simulink model "brine_3_1"  (R2018b)
settings: Solver=VariableStepAuto  StartTime=0.0  StopTime=10.0  RelTol=1e-3
settings Model: Creator=fyna  LastModifiedBy=fyna

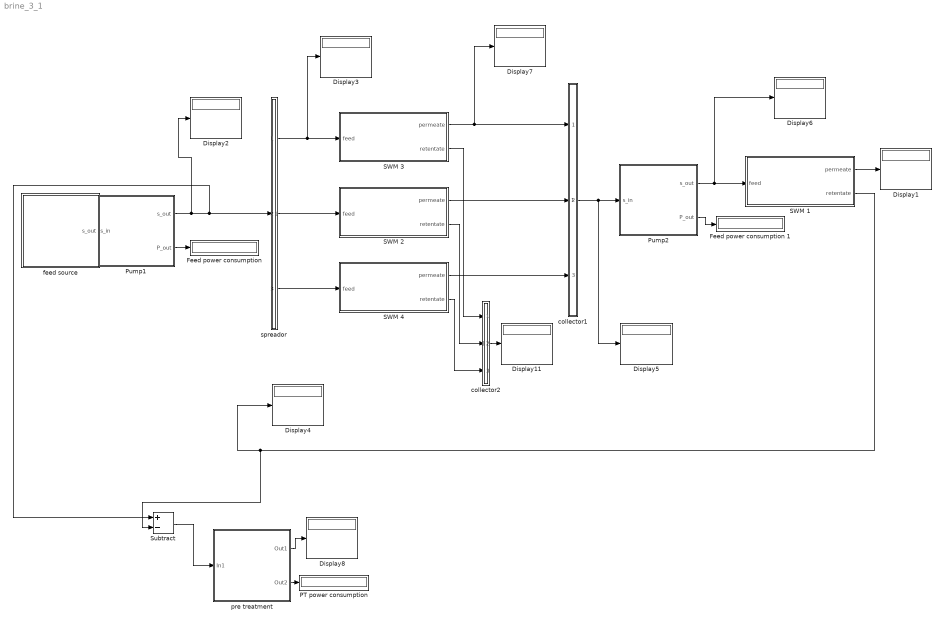
== system brine_3_1 ==
  Display{1..8,11} (9 alike) : Display
  "Feed power consumption " : Display
  Feed power consumption 1 : Display
  "PT power consumption " : Display
  Pump1 : Subsystem  mask(Hydraulic pump){p_f=100, eta=0.8}
      mask prompts: p_f "operating pressure [bar]"; eta "pump efficiency"
      mask help: The hydraulic pump pressurizes the incomming feed stream to the supplied operating pressure. It's power consumption is calculated as P = 3.6e-2*q*p/eta, [P] = kW.
      mask TypeOptions p_f:
      | operating pressure
      | /Value
      mask TypeOptions eta: efficiency/Value
      mask Display: image("pumpSymbol2.png")
  Pump2 : Subsystem  mask(Hydraulic pump){p_f=10, eta=0.8}
      mask prompts: p_f "operating pressure [bar]"; eta "pump efficiency"
      mask help: The hydraulic pump pressurizes the incomming feed stream to the supplied operating pressure. It's power consumption is calculated as P = 3.6e-2*q*p/eta, [P] = kW.
      mask TypeOptions p_f:
      | operating pressure
      | /Value
      mask TypeOptions eta: efficiency/Value
      mask Display: image("pumpSymbol2.png")
  SWM 1 : Subsystem  mask(8040 RO module){waterPerm=5, Value=0.995}
      mask prompts: waterPerm "water permeation coeff [lmh bar]]"; Value "salt rejection"
      mask help:
      | Reverse Osmosis module model. The permeate out-flow and feed out-flow are calculated from their respective in-flows and the membrane characteristics. A 28mil spacer is used in this module type.
      |
      | Input constants: membrane water permeability, salt rejection.
      mask TypeOptions waterPerm: waterPerm/Value
      mask TypeOptions Value: rejectionRate/Value
      mask Display: image('roSymbol.png');
  SWM 2 : Subsystem  mask(8040 RO module){waterPerm=5, Value=0.995}
      mask prompts: waterPerm "water permeation coeff [lmh bar]]"; Value "salt rejection"
      mask help:
      | Reverse Osmosis module model. The permeate out-flow and feed out-flow are calculated from their respective in-flows and the membrane characteristics. A 28mil spacer is used in this module type.
      |
      | Input constants: membrane water permeability, salt rejection.
      mask TypeOptions waterPerm: waterPerm/Value
      mask TypeOptions Value: rejectionRate/Value
      mask Display: image('roSymbol.png');
  SWM 3 : Subsystem  mask(8040 RO module){waterPerm=5, Value=0.995}
      mask prompts: waterPerm "water permeation coeff [lmh bar]]"; Value "salt rejection"
      mask help:
      | Reverse Osmosis module model. The permeate out-flow and feed out-flow are calculated from their respective in-flows and the membrane characteristics. A 28mil spacer is used in this module type.
      |
      | Input constants: membrane water permeability, salt rejection.
      mask TypeOptions waterPerm: waterPerm/Value
      mask TypeOptions Value: rejectionRate/Value
      mask Display: image('roSymbol.png');
  SWM 4 : Subsystem  mask(8040 RO module){waterPerm=5, Value=0.995}
      mask prompts: waterPerm "water permeation coeff [lmh bar]]"; Value "salt rejection"
      mask help:
      | Reverse Osmosis module model. The permeate out-flow and feed out-flow are calculated from their respective in-flows and the membrane characteristics. A 28mil spacer is used in this module type.
      |
      | Input constants: membrane water permeability, salt rejection.
      mask TypeOptions waterPerm: waterPerm/Value
      mask TypeOptions Value: rejectionRate/Value
      mask Display: image('roSymbol.png');
  Subtract : Sum  Inputs=+-
  collector1 : MATLAB Function  TreatAsAtomicUnit=on
  collector2 : MATLAB Function  TreatAsAtomicUnit=on
  feed source : Subsystem  mask(Feed source){Q=1.2e4, p=0, c=1.5}
      mask prompts: Q "flow rate Q [l/h]"; p "pressure p [bar]"; c "concentration c [mol/l]"
      mask help: This element is the starting point for the filtration system.
      mask TypeOptions Q: Q/Value
      mask TypeOptions p: p/Value
      mask TypeOptions c: c/Value
      mask Display: image('sourceSymbol.png');
  "pre treatment " : Subsystem  mask(Pre-treatment element){eta=0.8, k=1, A=100}
      mask prompts: eta "efficiency"; k "PT permeation coeff [m/(d bar)]"; A "PT membr area [m^2]"
      mask help: Simplified pre-treatment model for calculation of power demand only. The incoming stream is transfered to the outlet unchanged. From its flow rate, the pre-treatment pressure and the efficiency the power consumtion is calculated as: P = 3.6e-2*q*p/eta, [P] = kW.
      mask TypeOptions eta: nu/Value
      mask TypeOptions k: permeability const/Value
      mask TypeOptions A: membrSrf/Value
      mask Display: image('ptSymbol.png');
  spreador : MATLAB Function  TreatAsAtomicUnit=on
  wires:
  Pump1/2(P_out) -> "Feed power consumption "/1
  feed source/1(s_out) -> Pump1/1("s_in ")
  SWM 3/2(retentate) -> collector2/1(in_1)
  SWM 1/1(permeate) -> Display1/1
  Pump2/2(P_out) -> Feed power consumption 1/1
  Pump2/1(s_out) -> SWM 1/1(feed), Display6/1
  SWM 1/2(retentate) -> Subtract/2, Display4/1
  Pump1/1(s_out) -> Display2/1, Subtract/1, spreador/1(in_1)
  spreador/1(out_1) -> Display3/1, SWM 3/1(feed)
  spreador/2(data) -> SWM 2/1(feed)
  spreador/3(data1) -> SWM 4/1(feed)
  SWM 2/2(retentate) -> collector2/2(data)
  SWM 4/2(retentate) -> collector2/3(data1)
  SWM 3/1(permeate) -> Display7/1, collector1/1(in_1)
  SWM 4/1(permeate) -> collector1/3(data1)
  SWM 2/1(permeate) -> collector1/2(data)
  collector1/1(out_1) -> Pump2/1("s_in "), Display5/1
  collector2/1(out_1) -> Display11/1
  "pre treatment "/2(Out2) -> "PT power consumption "/1
  Subtract/1 -> "pre treatment "/1(In1)
  "pre treatment "/1(Out1) -> Display8/1

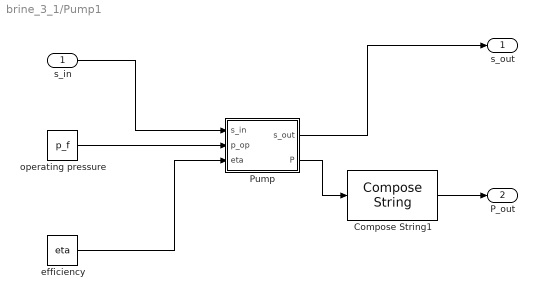
== system brine_3_1/Pump1 ==
  "s_in " : Inport
  Compose String1 : ComposeString  Format='P = %.3f kW'
  Pump : MATLAB Function  TreatAsAtomicUnit=on
  efficiency : Constant  Value=eta
  "operating pressure " : Constant  Value=p_f
  s_out : Outport
  P_out : Outport  Port=2
  wires:
  Pump/1(s_out) -> s_out/1
  efficiency/1 -> Pump/3(eta)
  Compose String1/1 -> P_out/1
  Pump/2(P) -> Compose String1/1
  "s_in "/1 -> Pump/1(s_in)
  "operating pressure "/1 -> Pump/2(p_op)

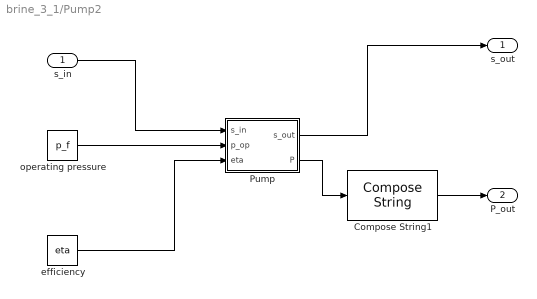
== system brine_3_1/Pump2 ==
  "s_in " : Inport
  Compose String1 : ComposeString  Format='P = %.3f kW'
  Pump : MATLAB Function  TreatAsAtomicUnit=on
  efficiency : Constant  Value=eta
  "operating pressure " : Constant  Value=p_f
  s_out : Outport
  P_out : Outport  Port=2
  wires:
  Pump/1(s_out) -> s_out/1
  efficiency/1 -> Pump/3(eta)
  Compose String1/1 -> P_out/1
  Pump/2(P) -> Compose String1/1
  "s_in "/1 -> Pump/1(s_in)
  "operating pressure "/1 -> Pump/2(p_op)

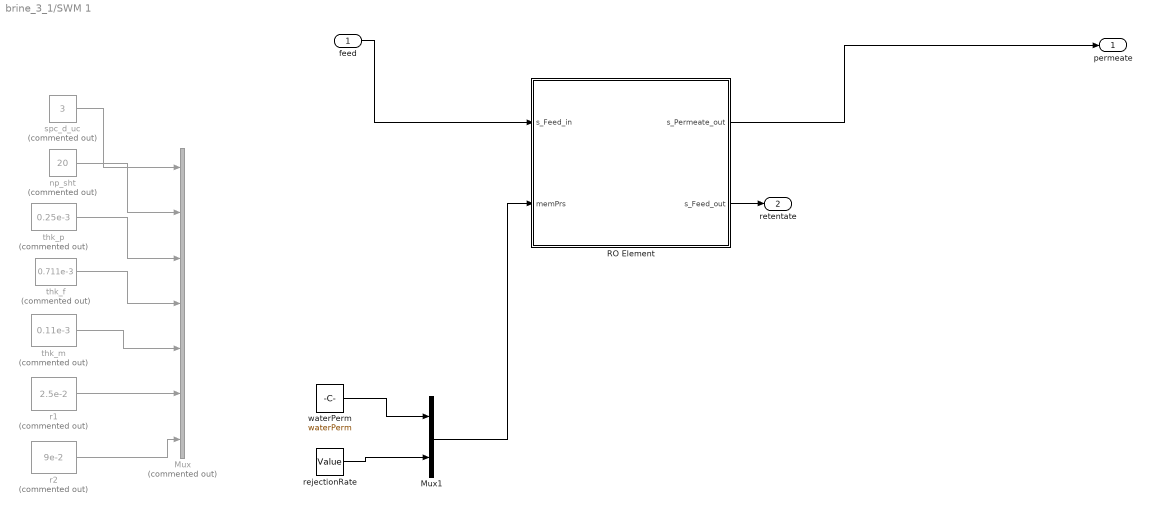
== system brine_3_1/SWM 1 ==
  feed : Inport
  Mux : Mux  Commented=on  Inputs=7
  Mux1 : Mux  Inputs=2
  RO Element : MATLAB Function  TreatAsAtomicUnit=on
  np_sht : Constant  Commented=on  Value=20
  r1 : Constant  Commented=on  Value=2.5e-2
  r2 : Constant  Commented=on  Value=9e-2
  rejectionRate : Constant  Value=Value
  spc_d_uc : Constant  Commented=on  Value=3
  thk_f : Constant  Commented=on  Value=0.711e-3
  thk_m : Constant  Commented=on  Value=0.11e-3
  thk_p : Constant  Commented=on  Value=0.25e-3
  waterPerm : Constant  Value=waterPerm
  permeate : Outport
  retentate : Outport  Port=2
  wires:
  spc_d_uc/1 -> Mux/1
  feed/1 -> RO Element/1(s_Feed_in)
  waterPerm/1 -> Mux1/1
  r1/1 -> Mux/6
  thk_m/1 -> Mux/5
  Mux1/1 -> RO Element/2(memPrs)
  r2/1 -> Mux/7
  RO Element/2(s_Feed_out) -> retentate/1
  rejectionRate/1 -> Mux1/2
  RO Element/1(s_Permeate_out) -> permeate/1
  thk_p/1 -> Mux/3
  thk_f/1 -> Mux/4
  np_sht/1 -> Mux/2

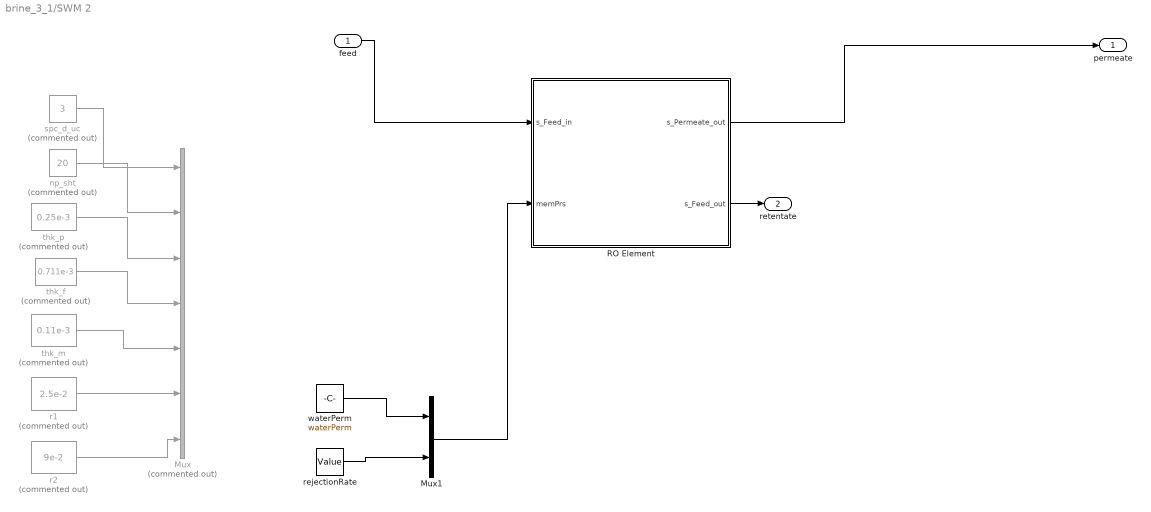
== system brine_3_1/SWM 2 ==
  feed : Inport
  Mux : Mux  Commented=on  Inputs=7
  Mux1 : Mux  Inputs=2
  RO Element : MATLAB Function  TreatAsAtomicUnit=on
  np_sht : Constant  Commented=on  Value=20
  r1 : Constant  Commented=on  Value=2.5e-2
  r2 : Constant  Commented=on  Value=9e-2
  rejectionRate : Constant  Value=Value
  spc_d_uc : Constant  Commented=on  Value=3
  thk_f : Constant  Commented=on  Value=0.711e-3
  thk_m : Constant  Commented=on  Value=0.11e-3
  thk_p : Constant  Commented=on  Value=0.25e-3
  waterPerm : Constant  Value=waterPerm
  permeate : Outport
  retentate : Outport  Port=2
  wires:
  spc_d_uc/1 -> Mux/1
  feed/1 -> RO Element/1(s_Feed_in)
  waterPerm/1 -> Mux1/1
  r1/1 -> Mux/6
  thk_m/1 -> Mux/5
  Mux1/1 -> RO Element/2(memPrs)
  r2/1 -> Mux/7
  RO Element/2(s_Feed_out) -> retentate/1
  rejectionRate/1 -> Mux1/2
  RO Element/1(s_Permeate_out) -> permeate/1
  thk_p/1 -> Mux/3
  thk_f/1 -> Mux/4
  np_sht/1 -> Mux/2

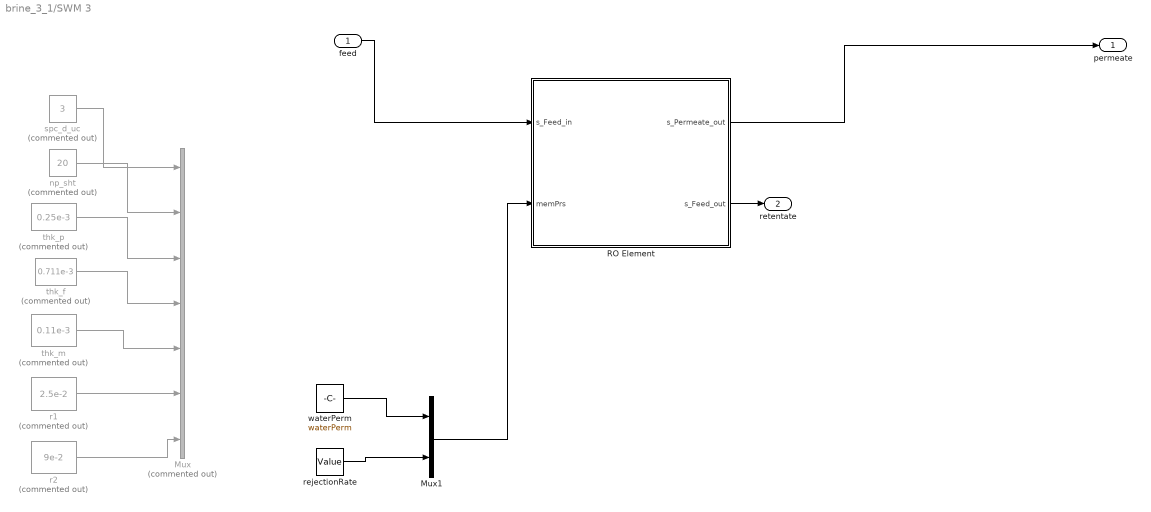
== system brine_3_1/SWM 3 ==
  feed : Inport
  Mux : Mux  Commented=on  Inputs=7
  Mux1 : Mux  Inputs=2
  RO Element : MATLAB Function  TreatAsAtomicUnit=on
  np_sht : Constant  Commented=on  Value=20
  r1 : Constant  Commented=on  Value=2.5e-2
  r2 : Constant  Commented=on  Value=9e-2
  rejectionRate : Constant  Value=Value
  spc_d_uc : Constant  Commented=on  Value=3
  thk_f : Constant  Commented=on  Value=0.711e-3
  thk_m : Constant  Commented=on  Value=0.11e-3
  thk_p : Constant  Commented=on  Value=0.25e-3
  waterPerm : Constant  Value=waterPerm
  permeate : Outport
  retentate : Outport  Port=2
  wires:
  spc_d_uc/1 -> Mux/1
  feed/1 -> RO Element/1(s_Feed_in)
  waterPerm/1 -> Mux1/1
  r1/1 -> Mux/6
  thk_m/1 -> Mux/5
  Mux1/1 -> RO Element/2(memPrs)
  r2/1 -> Mux/7
  RO Element/2(s_Feed_out) -> retentate/1
  rejectionRate/1 -> Mux1/2
  RO Element/1(s_Permeate_out) -> permeate/1
  thk_p/1 -> Mux/3
  thk_f/1 -> Mux/4
  np_sht/1 -> Mux/2

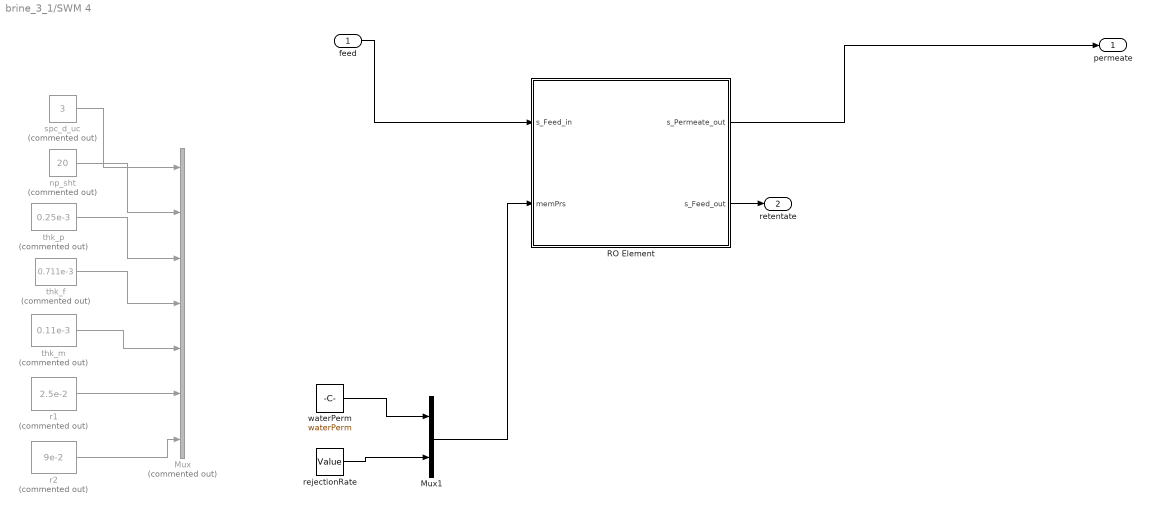
== system brine_3_1/SWM 4 ==
  feed : Inport
  Mux : Mux  Commented=on  Inputs=7
  Mux1 : Mux  Inputs=2
  RO Element : MATLAB Function  TreatAsAtomicUnit=on
  np_sht : Constant  Commented=on  Value=20
  r1 : Constant  Commented=on  Value=2.5e-2
  r2 : Constant  Commented=on  Value=9e-2
  rejectionRate : Constant  Value=Value
  spc_d_uc : Constant  Commented=on  Value=3
  thk_f : Constant  Commented=on  Value=0.711e-3
  thk_m : Constant  Commented=on  Value=0.11e-3
  thk_p : Constant  Commented=on  Value=0.25e-3
  waterPerm : Constant  Value=waterPerm
  permeate : Outport
  retentate : Outport  Port=2
  wires:
  spc_d_uc/1 -> Mux/1
  feed/1 -> RO Element/1(s_Feed_in)
  waterPerm/1 -> Mux1/1
  r1/1 -> Mux/6
  thk_m/1 -> Mux/5
  Mux1/1 -> RO Element/2(memPrs)
  r2/1 -> Mux/7
  RO Element/2(s_Feed_out) -> retentate/1
  rejectionRate/1 -> Mux1/2
  RO Element/1(s_Permeate_out) -> permeate/1
  thk_p/1 -> Mux/3
  thk_f/1 -> Mux/4
  np_sht/1 -> Mux/2

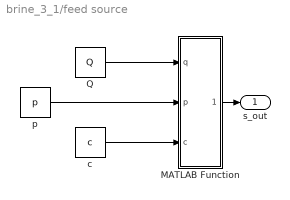
== system brine_3_1/feed source ==
  MATLAB Function : MATLAB Function  TreatAsAtomicUnit=on
  Q : Constant  Value=Q
  c : Constant  Value=c
  p : Constant  Value=p
  s_out : Outport
  wires:
  MATLAB Function/1(s_out) -> s_out/1
  c/1 -> MATLAB Function/3(c)
  p/1 -> MATLAB Function/2(p)
  Q/1 -> MATLAB Function/1(q)

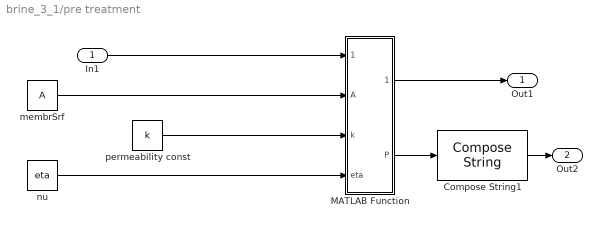
== system brine_3_1/pre treatment  ==
  In1 : Inport
  Compose String1 : ComposeString  Format='P = %.3f kW'
  MATLAB Function : MATLAB Function  TreatAsAtomicUnit=on
  membrSrf : Constant  Value=A
  nu : Constant  Value=eta
  permeability const : Constant  Value=k
  Out1 : Outport
  Out2 : Outport  Port=2
  wires:
  MATLAB Function/1(s_out) -> Out1/1
  In1/1 -> MATLAB Function/1(s_in)
  membrSrf/1 -> MATLAB Function/2(A)
  nu/1 -> MATLAB Function/4(eta)
  MATLAB Function/2(P) -> Compose String1/1
  Compose String1/1 -> Out2/1
  permeability const/1 -> MATLAB Function/3(k)

== matlab function brine_3_1/SWM 1/RO Element ==
  data: s_Feed_in input; s_Permeate_out output; s_Feed_out output; memPrs input
function [s_Permeate_out, s_Feed_out] = fcn(s_Feed_in, memPrs)

% moduleParas = [d_uc, no_sht, thk_d, thk_f, thk_m, r1, r2]

r_fl    = 2.5e-4;
h_ch    = 7.11e-4;
l_f     = 2.822e-3;
eps     = 1.0 - (3.14*r_fl^2*2.0)/(l_f*h_ch);

% ---------------------------------fixing flow rate:
nbSheets = 20;
l_s     = 1.1;
l_l     = 0.93;

q_in    = s_Feed_in(1)/3.6*1e-6;        %m^3/s
U       = q_in/(l_s*0.711e-3*nbSheets);

dh      = 1.0673e-3;        % m
re      = U*dh*1e6;
% sh      = 4.43655*re^0.48267

k_dc    = 1.654*(2.0*r_fl/h_ch)^-0.039*eps^0.75*0.7071^0.086;
sc      = 690;
sh     = 0.664*k_dc*re^0.5*sc^0.33*(dh/l_f)^0.5;

D       = 1.45e-9;          % m^2/s
k_m     = sh*D/dh;        

A_m     = memPrs(1)/3.6*1e-11;  % m/s/pa
zeta    = 8.05e4;               % pa m^3/kg
molarMassNaCl   = 58.44276;     % g/mol
c_f     = s_Feed_in(3)*molarMassNaCl;       %g/l
d_p     = s_Feed_in(2)*1e5;  % pa

a   = 0.0;
b   = 1e-4;

presDiff = d_p - c_f*zeta;
if presDiff > 0
    %fprintf('pi_f = %e, p_f = %e\n',c_f*zeta, d_p);
    jw_uc   = 0.0;
    while abs(a-b) > 1e-10
        x   = 0.5*(a+b);
        fa  = a - A_m*(  d_p - zeta*( c_f*exp(a/k_m) )  );
        fx  = x - A_m*(  d_p - zeta*( c_f*exp(x/k_m) )  );
%         fprintf('a = %e, b = %e, x = %e, abs(a-b) = %e\n',a,b,x, abs(a-b));

        if fa*fx>0
            a   = x;
        else
            b   = x;
        end
    end
    jw_uc   = 0.5*(a+b);
else
    fprintf('osmotic pressure higher than feed hydraulic pressure: pi_f = %e, p_f = %e\n',c_f*zeta, d_p);
    jw_uc   = 0.0;
end

% fprintf('jw = %e\n',jw_uc);
% n_s = round(l_s/(2.822e-3));
% n_l = round(l_l/(2.822e-3));
% area_uc = 16e-6;                %m^2
% area_mod = area_uc*n_s*n_l*nbSheets

area_mod = l_s*l_l*2*nbSheets;

q_mem = area_mod*jw_uc;         % m^3/s
if q_mem > q_in
    q_mem = q_in;
end

% ---------------------------------fixing solute flux:
R_m   = memPrs(2);
q_s_m = q_mem*c_f*(1.0-R_m);    % kg/m^3, solute mass flow rate through membrane
q_s_r = (q_in*c_f - q_s_m);     % kg/m^3, solute mass flow rate retained in feed channel

% ---------------------------------fixing pressure drop:
% f       = 22.91*re^-0.606
f      = 6.23*re^-0.3;
dP      = f*U^2*1e3*l_l/(2.0*dh)*1e-5;  % bar
% fprintf('f = %e\n',area_mod);

q_feed_out = (q_in-q_mem)*3.6e6 ;
p_feed_out = s_Feed_in(2) - dP;q_perm_out = q_mem*3.6e6;      %l/h
c_feed_out = q_s_r/(q_feed_out/3.6e6)/molarMassNaCl;

q_perm_out = q_mem*3.6e6;      %l/h
p_perm_out = 0;

if q_mem > 0
    c_perm_out =  q_s_m/q_mem/molarMassNaCl;
else
    c_perm_out = 0;
end

s_Feed_out      = [q_feed_out, p_feed_out, c_feed_out];
s_Permeate_out  = [q_perm_out, p_perm_out, c_perm_out];

== matlab function brine_3_1/Pump2/Pump ==
  data: s_in input; p_op input; s_out output; eta input; P output
function [s_out,P ] = fcn(s_in, p_op, eta)
q = s_in(1);
dp = p_op - s_in(2);
P = q*dp/eta/3.6e4;     % power consumption in kW
s_out = [q,p_op,s_in(3)];

== matlab function brine_3_1/Pump1/Pump ==
  data: s_in input; p_op input; s_out output; eta input; P output
function [s_out,P ] = fcn(s_in, p_op, eta)
q = s_in(1);
dp = p_op - s_in(2);
P = q*dp/eta/3.6e4;     % power consumption in kW
s_out = [q,p_op,s_in(3)];

== matlab function brine_3_1/SWM 3/RO Element ==
  data: s_Feed_in input; s_Permeate_out output; s_Feed_out output; memPrs input
function [s_Permeate_out, s_Feed_out] = fcn(s_Feed_in, memPrs)

% moduleParas = [d_uc, no_sht, thk_d, thk_f, thk_m, r1, r2]

r_fl    = 2.5e-4;
h_ch    = 7.11e-4;
l_f     = 2.822e-3;
eps     = 1.0 - (3.14*r_fl^2*2.0)/(l_f*h_ch);

% ---------------------------------fixing flow rate:
nbSheets = 20;
l_s     = 1.1;
l_l     = 0.93;

q_in    = s_Feed_in(1)/3.6*1e-6;        %m^3/s
U       = q_in/(l_s*0.711e-3*nbSheets);

dh      = 1.0673e-3;        % m
re      = U*dh*1e6;
% sh      = 4.43655*re^0.48267

k_dc    = 1.654*(2.0*r_fl/h_ch)^-0.039*eps^0.75*0.7071^0.086;
sc      = 690;
sh     = 0.664*k_dc*re^0.5*sc^0.33*(dh/l_f)^0.5;

D       = 1.45e-9;          % m^2/s
k_m     = sh*D/dh;        

A_m     = memPrs(1)/3.6*1e-11;  % m/s/pa
zeta    = 8.05e4;               % pa m^3/kg
molarMassNaCl   = 58.44276;     % g/mol
c_f     = s_Feed_in(3)*molarMassNaCl;       %g/l
d_p     = s_Feed_in(2)*1e5;  % pa

a   = 0.0;
b   = 1e-4;

presDiff = d_p - c_f*zeta;
if presDiff > 0
    %fprintf('pi_f = %e, p_f = %e\n',c_f*zeta, d_p);
    jw_uc   = 0.0;
    while abs(a-b) > 1e-10
        x   = 0.5*(a+b);
        fa  = a - A_m*(  d_p - zeta*( c_f*exp(a/k_m) )  );
        fx  = x - A_m*(  d_p - zeta*( c_f*exp(x/k_m) )  );
%         fprintf('a = %e, b = %e, x = %e, abs(a-b) = %e\n',a,b,x, abs(a-b));

        if fa*fx>0
            a   = x;
        else
            b   = x;
        end
    end
    jw_uc   = 0.5*(a+b);
else
    fprintf('osmotic pressure higher than feed hydraulic pressure: pi_f = %e, p_f = %e\n',c_f*zeta, d_p);
    jw_uc   = 0.0;
end

% fprintf('jw = %e\n',jw_uc);
% n_s = round(l_s/(2.822e-3));
% n_l = round(l_l/(2.822e-3));
% area_uc = 16e-6;                %m^2
% area_mod = area_uc*n_s*n_l*nbSheets

area_mod = l_s*l_l*2*nbSheets;

q_mem = area_mod*jw_uc;         % m^3/s
if q_mem > q_in
    q_mem = q_in;
end

% ---------------------------------fixing solute flux:
R_m   = memPrs(2);
q_s_m = q_mem*c_f*(1.0-R_m);    % kg/m^3, solute mass flow rate through membrane
q_s_r = (q_in*c_f - q_s_m);     % kg/m^3, solute mass flow rate retained in feed channel

% ---------------------------------fixing pressure drop:
% f       = 22.91*re^-0.606
f      = 6.23*re^-0.3;
dP      = f*U^2*1e3*l_l/(2.0*dh)*1e-5;  % bar
% fprintf('f = %e\n',area_mod);

q_feed_out = (q_in-q_mem)*3.6e6 ;
p_feed_out = s_Feed_in(2) - dP;q_perm_out = q_mem*3.6e6;      %l/h
c_feed_out = q_s_r/(q_feed_out/3.6e6)/molarMassNaCl;

q_perm_out = q_mem*3.6e6;      %l/h
p_perm_out = 0;

if q_mem > 0
    c_perm_out =  q_s_m/q_mem/molarMassNaCl;
else
    c_perm_out = 0;
end

s_Feed_out      = [q_feed_out, p_feed_out, c_feed_out];
s_Permeate_out  = [q_perm_out, p_perm_out, c_perm_out];

== matlab function brine_3_1/SWM 2/RO Element ==
  data: s_Feed_in input; s_Permeate_out output; s_Feed_out output; memPrs input
function [s_Permeate_out, s_Feed_out] = fcn(s_Feed_in, memPrs)

% moduleParas = [d_uc, no_sht, thk_d, thk_f, thk_m, r1, r2]

r_fl    = 2.5e-4;
h_ch    = 7.11e-4;
l_f     = 2.822e-3;
eps     = 1.0 - (3.14*r_fl^2*2.0)/(l_f*h_ch);

% ---------------------------------fixing flow rate:
nbSheets = 20;
l_s     = 1.1;
l_l     = 0.93;

q_in    = s_Feed_in(1)/3.6*1e-6;        %m^3/s
U       = q_in/(l_s*0.711e-3*nbSheets);

dh      = 1.0673e-3;        % m
re      = U*dh*1e6;
% sh      = 4.43655*re^0.48267

k_dc    = 1.654*(2.0*r_fl/h_ch)^-0.039*eps^0.75*0.7071^0.086;
sc      = 690;
sh     = 0.664*k_dc*re^0.5*sc^0.33*(dh/l_f)^0.5;

D       = 1.45e-9;          % m^2/s
k_m     = sh*D/dh;        

A_m     = memPrs(1)/3.6*1e-11;  % m/s/pa
zeta    = 8.05e4;               % pa m^3/kg
molarMassNaCl   = 58.44276;     % g/mol
c_f     = s_Feed_in(3)*molarMassNaCl;       %g/l
d_p     = s_Feed_in(2)*1e5;  % pa

a   = 0.0;
b   = 1e-4;

presDiff = d_p - c_f*zeta;
if presDiff > 0
    %fprintf('pi_f = %e, p_f = %e\n',c_f*zeta, d_p);
    jw_uc   = 0.0;
    while abs(a-b) > 1e-10
        x   = 0.5*(a+b);
        fa  = a - A_m*(  d_p - zeta*( c_f*exp(a/k_m) )  );
        fx  = x - A_m*(  d_p - zeta*( c_f*exp(x/k_m) )  );
%         fprintf('a = %e, b = %e, x = %e, abs(a-b) = %e\n',a,b,x, abs(a-b));

        if fa*fx>0
            a   = x;
        else
            b   = x;
        end
    end
    jw_uc   = 0.5*(a+b);
else
    fprintf('osmotic pressure higher than feed hydraulic pressure: pi_f = %e, p_f = %e\n',c_f*zeta, d_p);
    jw_uc   = 0.0;
end

% fprintf('jw = %e\n',jw_uc);
% n_s = round(l_s/(2.822e-3));
% n_l = round(l_l/(2.822e-3));
% area_uc = 16e-6;                %m^2
% area_mod = area_uc*n_s*n_l*nbSheets

area_mod = l_s*l_l*2*nbSheets;

q_mem = area_mod*jw_uc;         % m^3/s
if q_mem > q_in
    q_mem = q_in;
end

% ---------------------------------fixing solute flux:
R_m   = memPrs(2);
q_s_m = q_mem*c_f*(1.0-R_m);    % kg/m^3, solute mass flow rate through membrane
q_s_r = (q_in*c_f - q_s_m);     % kg/m^3, solute mass flow rate retained in feed channel

% ---------------------------------fixing pressure drop:
% f       = 22.91*re^-0.606
f      = 6.23*re^-0.3;
dP      = f*U^2*1e3*l_l/(2.0*dh)*1e-5;  % bar
% fprintf('f = %e\n',area_mod);

q_feed_out = (q_in-q_mem)*3.6e6 ;
p_feed_out = s_Feed_in(2) - dP;q_perm_out = q_mem*3.6e6;      %l/h
c_feed_out = q_s_r/(q_feed_out/3.6e6)/molarMassNaCl;

q_perm_out = q_mem*3.6e6;      %l/h
p_perm_out = 0;

if q_mem > 0
    c_perm_out =  q_s_m/q_mem/molarMassNaCl;
else
    c_perm_out = 0;
end

s_Feed_out      = [q_feed_out, p_feed_out, c_feed_out];
s_Permeate_out  = [q_perm_out, p_perm_out, c_perm_out];

== matlab function brine_3_1/SWM 4/RO Element ==
  data: s_Feed_in input; s_Permeate_out output; s_Feed_out output; memPrs input
function [s_Permeate_out, s_Feed_out] = fcn(s_Feed_in, memPrs)

% moduleParas = [d_uc, no_sht, thk_d, thk_f, thk_m, r1, r2]

r_fl    = 2.5e-4;
h_ch    = 7.11e-4;
l_f     = 2.822e-3;
eps     = 1.0 - (3.14*r_fl^2*2.0)/(l_f*h_ch);

% ---------------------------------fixing flow rate:
nbSheets = 20;
l_s     = 1.1;
l_l     = 0.93;

q_in    = s_Feed_in(1)/3.6*1e-6;        %m^3/s
U       = q_in/(l_s*0.711e-3*nbSheets);

dh      = 1.0673e-3;        % m
re      = U*dh*1e6;
% sh      = 4.43655*re^0.48267

k_dc    = 1.654*(2.0*r_fl/h_ch)^-0.039*eps^0.75*0.7071^0.086;
sc      = 690;
sh     = 0.664*k_dc*re^0.5*sc^0.33*(dh/l_f)^0.5;

D       = 1.45e-9;          % m^2/s
k_m     = sh*D/dh;        

A_m     = memPrs(1)/3.6*1e-11;  % m/s/pa
zeta    = 8.05e4;               % pa m^3/kg
molarMassNaCl   = 58.44276;     % g/mol
c_f     = s_Feed_in(3)*molarMassNaCl;       %g/l
d_p     = s_Feed_in(2)*1e5;  % pa

a   = 0.0;
b   = 1e-4;

presDiff = d_p - c_f*zeta;
if presDiff > 0
    %fprintf('pi_f = %e, p_f = %e\n',c_f*zeta, d_p);
    jw_uc   = 0.0;
    while abs(a-b) > 1e-10
        x   = 0.5*(a+b);
        fa  = a - A_m*(  d_p - zeta*( c_f*exp(a/k_m) )  );
        fx  = x - A_m*(  d_p - zeta*( c_f*exp(x/k_m) )  );
%         fprintf('a = %e, b = %e, x = %e, abs(a-b) = %e\n',a,b,x, abs(a-b));

        if fa*fx>0
            a   = x;
        else
            b   = x;
        end
    end
    jw_uc   = 0.5*(a+b);
else
    fprintf('osmotic pressure higher than feed hydraulic pressure: pi_f = %e, p_f = %e\n',c_f*zeta, d_p);
    jw_uc   = 0.0;
end

% fprintf('jw = %e\n',jw_uc);
% n_s = round(l_s/(2.822e-3));
% n_l = round(l_l/(2.822e-3));
% area_uc = 16e-6;                %m^2
% area_mod = area_uc*n_s*n_l*nbSheets

area_mod = l_s*l_l*2*nbSheets;

q_mem = area_mod*jw_uc;         % m^3/s
if q_mem > q_in
    q_mem = q_in;
end

% ---------------------------------fixing solute flux:
R_m   = memPrs(2);
q_s_m = q_mem*c_f*(1.0-R_m);    % kg/m^3, solute mass flow rate through membrane
q_s_r = (q_in*c_f - q_s_m);     % kg/m^3, solute mass flow rate retained in feed channel

% ---------------------------------fixing pressure drop:
% f       = 22.91*re^-0.606
f      = 6.23*re^-0.3;
dP      = f*U^2*1e3*l_l/(2.0*dh)*1e-5;  % bar
% fprintf('f = %e\n',area_mod);

q_feed_out = (q_in-q_mem)*3.6e6 ;
p_feed_out = s_Feed_in(2) - dP;q_perm_out = q_mem*3.6e6;      %l/h
c_feed_out = q_s_r/(q_feed_out/3.6e6)/molarMassNaCl;

q_perm_out = q_mem*3.6e6;      %l/h
p_perm_out = 0;

if q_mem > 0
    c_perm_out =  q_s_m/q_mem/molarMassNaCl;
else
    c_perm_out = 0;
end

s_Feed_out      = [q_feed_out, p_feed_out, c_feed_out];
s_Permeate_out  = [q_perm_out, p_perm_out, c_perm_out];

== matlab function brine_3_1/collector1 ==
  data: in_1 input; out_1 output; data input; data1 input
function out_1  = fork(in_1, data, data1)
% reducing all input streams to one stream

switch nargin
    case 1
        sInAr = in_1;
    case 2
        sInAr = [data; in_1];
    case 3
        sInAr = [data; data1; in_1];
    case 4
        sInAr = [data; data1; data2; in_1];
    case 5
        sInAr = [data; data1; data2; data3; in_1];
    case 6
        sInAr = [data; data1; data2; data3; data4; in_1];
    case 7
        sInAr = [data; data1; data2; data3; data4; data5; in_1];
    case 8
        sInAr = [data; data1; data2; data3; data4; data5; data6; in_1];
    case 9
        sInAr = [data; data1; data2; data3; data4; data5; data6; data7; in_1];
    case 10
        sInAr = [data; data1; data2; data3; data4; data5; data6; data7; data8; in_1];
    otherwise
        fprintf("no input stream\n");
end

q_sum = 0;
c_avg = 0;
p_sum = 0;
[m,n] = size(sInAr); % m: nb rows (incoming data) n: nb of columns (3)

for i=1:m
   q_sum = q_sum + sInAr(i,1);
   c_avg = c_avg + sInAr(i,1)*sInAr(i,3);
end
c_avg = c_avg/q_sum;

out_1 = [q_sum, sInAr(1,2), c_avg];

== matlab function brine_3_1/collector2 ==
  data: in_1 input; out_1 output; data input; data1 input
function out_1  = fork(in_1, data, data1)
% reducing all input streams to one stream

switch nargin
    case 1
        sInAr = in_1;
    case 2
        sInAr = [data; in_1];
    case 3
        sInAr = [data; data1; in_1];
    case 4
        sInAr = [data; data1; data2; in_1];
    case 5
        sInAr = [data; data1; data2; data3; in_1];
    case 6
        sInAr = [data; data1; data2; data3; data4; in_1];
    case 7
        sInAr = [data; data1; data2; data3; data4; data5; in_1];
    case 8
        sInAr = [data; data1; data2; data3; data4; data5; data6; in_1];
    case 9
        sInAr = [data; data1; data2; data3; data4; data5; data6; data7; in_1];
    case 10
        sInAr = [data; data1; data2; data3; data4; data5; data6; data7; data8; in_1];
    otherwise
        fprintf("no input stream\n");
end

q_sum = 0;
c_avg = 0;
p_sum = 0;
[m,n] = size(sInAr); % m: nb rows (incoming data) n: nb of columns (3)

for i=1:m
   q_sum = q_sum + sInAr(i,1);
   c_avg = c_avg + sInAr(i,1)*sInAr(i,3);
end
c_avg = c_avg/q_sum;

out_1 = [q_sum, sInAr(1,2), c_avg];

== matlab function brine_3_1/feed source/MATLAB Function ==
  data: q input; s_out output; p input; c input
function s_out = fcn(q,p,c)
s_out = [q,p,c];

== matlab function brine_3_1/pre treatment /MATLAB Function ==
  data: s_in input; A input; k input; eta input; s_out output; P output
function [s_out,P ] = pt(s_in, A, k, eta)
q = s_in(1)*1e-6/3.6; % m^3/s
dp = q/(k/(8.64e9)*A);  % Pa
P = q*dp*1e-3/eta;     % power consumption in kW
s_out = s_in;

== matlab function brine_3_1/spreador ==
  data: in_1 input; out_1 output; data output; data1 output
function [out_1, data, data1] = fork(in_1)
% spreading one input stream to several output streams

switch nargout
    case 1
        out_1 = in_1;
    case 2
        out_1 = [in_1(1)/nargout, in_1(2), in_1(3)];
        data  = out_1;
    case 3
        out_1 = [in_1(1)/nargout, in_1(2), in_1(3)];
        data  = out_1;
        data1  = out_1;
    case 4
        out_1 = [in_1(1)/nargout, in_1(2), in_1(3)];
        data  = out_1;
        data1  = out_1;
        data2  = out_1;
    case 5
        out_1 = [in_1(1)/nargout, in_1(2), in_1(3)];
        data  = out_1;
        data1  = out_1;
        data2  = out_1;
        data3  = out_1;
    case 6
        out_1 = [in_1(1)/nargout, in_1(2), in_1(3)];
        data  = out_1;
        data1  = out_1;
        data2  = out_1;
        data3  = out_1;
        data4  = out_1;
    case 7
        out_1 = [in_1(1)/nargout, in_1(2), in_1(3)];
        data  = out_1;
        data1  = out_1;
        data2  = out_1;
        data3  = out_1;
        data4  = out_1;
        data5  = out_1;
    case 8
        out_1 = [in_1(1)/nargout, in_1(2), in_1(3)];
        data  = out_1;
        data1  = out_1;
        data2  = out_1;
        data3  = out_1;
        data4  = out_1;
        data5  = out_1;
        data6  = out_1;
    case 9
        out_1 = [in_1(1)/nargout, in_1(2), in_1(3)];
        data  = out_1;
        data1  = out_1;
        data2  = out_1;
        data3  = out_1;
        data4  = out_1;
        data5  = out_1;
        data6  = out_1;
        data7  = out_1;
    case 10
        out_1 = [in_1(1)/nargout, in_1(2), in_1(3)];
        data  = out_1;
        data1  = out_1;
        data2  = out_1;
        data3  = out_1;
        data4  = out_1;
        data5  = out_1;
        data6  = out_1;
        data7  = out_1;
        data8  = out_1;
    otherwise
        fprintf("no input stream\n");
end
